simulink model "sldemo_fuelsys"  (R2024a)
settings: Solver=ode45  StartTime=0  StopTime=2000  FixedStep=0.001  RelTol=1e-5  AbsTol=1e-6
PostLoadFcn:
  | sldemo_fuelsys_data(bdroot,'initialize_data','orig','float');
model workspace (MAT data in the model file):
  PressEst = [0.806253176324 0.553142316929 0.37151500209 0.277667903103 0.220198954207 0.181288665766 0.153200000489 0.115431020872 0.0913067476324 0.0746519188607 0.0625231108324 0.0533383634277 ... (306 elements, 18x17)]
  PressVect = [0.05 0.1 0.15 0.2 0.25 0.3 0.35 0.4 0.45 0.5 0.55 0.6 ... (19 elements, 1x19)]
  PumpCon = [-0.0556348 -0.0022828 0.0256932 0.0435188 0.0562692 0.0661194857143 0.0741572 0.08697 0.0972452 0.106070342857 0.1139892 0.121303866667 ... (342 elements, 18x19)]
  RampRateKiX = [100 200 300 400 500 600]
  RampRateKiY = [0 0.2 0.4 0.6 0.8 1]
  RampRateKiZ = [0.012 0.024 0.036 0.048 0.06 0.072 0.024 0.048 0.072 0.096 0.12 0.144 ... (36 elements, 6x6)]
  SpeedEst = [471.837839721 550.80940091 777.559313277 1080.9243499 1418.36795322 1769.7468768 2125.37309264 2480.20345067 2831.37796793 3177.14006959 3516.32917143 4064.90417867 ... (323 elements, 17x19)]
  SpeedVect = [50 75 100 125 150 175 200 250 300 350 400 450 ... (18 elements, 1x18)]
  ThrotEst = [0 0 0 0 0 0 0 0 0 0 0 0 ... (342 elements, 18x19)]
  ThrotVect = [0 3 6 9 12 15 18 21 24 27 30 35 ... (17 elements, 1x17)]
  ego_sw = 1
  engine_speed = 300
  hys = 25
  map_sw = 1
  max_ego = 1.2
  max_press = 0.95
  max_speed = 628
  max_throt = 90
  min_press = 0.05
  min_speed = 50
  min_throt = 3
  speed_sw = 1
  st_range = 0.0001
  throttle_sw = 1
  zero_thresh = 250
undefined symbols (not defined in the file or in its folder): DiscIntNeverNeededParam, sld_FuelModes, sldvsubsys
libraries: simulink x4, simulink_extras x1
(part 2 of 2)

== system sldemo_fuelsys/fuel_rate_control/fuel_calc/switchable_compensation/disabled_mode ==
  note: Disabled Mode Fuel Mode
  Action Port : ActionPort  ActionPortLabel=default:
  shutoff : Constant  Value=0  OutDataTypeStr=Inherit: Inherit via back propagation
  fuel_rate : Outport  InitialOutput=0  VectorParamsAs1DForOutWhenUnconnected=off
  wires:
  shutoff/1 -> fuel_rate/1

== system sldemo_fuelsys/fuel_rate_control/fuel_calc/switchable_compensation/low_mode ==
  note: Low Mode Fuel Mode
  fb_correction : Inport
  ff_fuel_rate : Inport  Port=2
  Action Port : ActionPort  ActionPortLabel=case [ LOW ]:
  Discrete Filter : DiscreteFilter  Numerator=[8.7696 -8.5104]  Denominator=[1 -0.7408]  a0EqualsOne=on  RndMeth=Simplest  OutDataTypeStr=Inherit: Same as input
  Sum3 : Sum  OutDataTypeStr=s16En7  RndMeth=Simplest
  fuel_rate : Outport  InitialOutput=0  VectorParamsAs1DForOutWhenUnconnected=off
  wires:
  ff_fuel_rate/1 -> Sum3/2
  Discrete Filter/1 -> Sum3/1
  Sum3/1 -> fuel_rate/1
  fb_correction/1 -> Discrete Filter/1

== system sldemo_fuelsys/fuel_rate_control/fuel_calc/switchable_compensation/rich_mode ==
  note: Rich Mode Fuel Mode
  ff_fuel_rate : Inport
  fb_correction : Inport  Port=2
  Action Port : ActionPort  ActionPortLabel=case [ RICH ]:
  Discrete Filter : DiscreteFilter  Numerator=[0 0.2592]  Denominator=[1 -0.7408]  a0EqualsOne=on  RndMeth=Simplest  OutDataTypeStr=Inherit: Same as input
  Sum2 : Sum  OutDataTypeStr=s16En7  RndMeth=Simplest
  fuel_rate : Outport  InitialOutput=0  VectorParamsAs1DForOutWhenUnconnected=off
  wires:
  fb_correction/1 -> Sum2/2
  ff_fuel_rate/1 -> Sum2/1
  Sum2/1 -> Discrete Filter/1
  Discrete Filter/1 -> fuel_rate/1

== stateflow chart sldemo_fuelsys/fuel_rate_control/control_logic ==
  state O2 [parallel]
    settings: executionOrder=1  description=This state determines the validity of the exhaust gas oxygen sensor (EGO) data.
    state A
      du:
      es_o.ego = es_i.ego;
      state O2_warmup
        settings: description=The EGO sensor must come up to temperature before its data is reliable.
      state O2_normal
        settings: description=Normal EGO sensor operation gives a reliable indication of excess oxygen in the exhaust gas, from which air/fuel mixture can be inferred.
      state O2_failure
        settings: description=The EGO sensor has failed.
      (default) -> O2_warmup
      O2_warmup -> O2_normal : [after(480,tick)]
        settings: description=The value for sufficient warm up to operational temperature (nominally 4.8 seconds).
      O2_failure -> O2_normal : [es_i.ego < max_ego] / Fail.DEC;
      O2_normal -> O2_failure : [es_i.ego > max_ego] / Fail.INC;
        settings: description=The failure condition is indicated by excessive output voltage.
    (default) -> A
  state Pressure [parallel]
    settings: executionOrder=2  description=This state assesses the validity of the manifold absolute pressure (MAP) sensor.
    state normal
      du:
      es_o.map = es_i.map;
      settings: description=The manifold pressure sensor gives a reliable indication of absolute pressure (MAP).
    state fail
      du:
      es_o.map = map_estimate(es_i.speed, es_i.throttle);
      settings: description=The pressure sensor (manifold, or MAP) no longer produces reliable data.
    state map = map_estimate(speed, throttle) [function]
    (default) -> Pressure.normal
    Pressure.fail -> Pressure.normal : [es_i.map > min_press & ...
        | es_i.map < max_press] /
        | Fail.DEC;
    Pressure.normal -> Pressure.fail : [es_i.map > max_press | ...
        | es_i.map < min_press] /
        | Fail.INC;
  state Throttle [parallel]
    settings: executionOrder=3  description=This state determines the validity of the throttle sensor signal.
    state normal
      du:
      es_o.throttle = es_i.throttle;
      settings: description=The throttle sensor gives a reliable indication of the angle of the throttle plate.
    state fail
      du:
      es_o.throttle = throttle_estimate(es_i.speed,es_i.map);
      settings: description=Signal levels indicate that the throttle sensor data is no longer valid.
    state throttle = throttle_estimate(speed, map) [function]
    (default) -> Throttle.normal
    Throttle.fail -> Throttle.normal : [es_i.throttle >  min_throt & ...
        | es_i.throttle < max_throt] /
        | Fail.DEC;
    Throttle.normal -> Throttle.fail : [es_i.throttle> max_throt | ...
        | es_i.throttle < min_throt] /
        | Fail.INC;
      settings: description=A failure is indicated by data which is outside the expected range, typically due to an open or short circuit.
  state Speed [parallel]
    settings: executionOrder=4  description="This state infers the validity of the speed sensor data.  A failure is indicated by the presence of manifold vacuum at zero speed."
    state normal
      du:
      es_o.speed = es_i.speed;
      settings: description=The speed sensor data accurately represents the engine speed.
    state fail
      du:
      es_o.speed = speed_estimate(es_i.throttle, es_i.map);
      settings: description=The engine speed data is no longer available.
    state speed = speed_estimate(throttle, map) [function]
    (default) -> Speed.normal
    Speed.fail -> Speed.normal : [es_i.speed > 0C] /
        | Fail.DEC;
    Speed.normal -> Speed.fail : [es_i.speed == 0C & ...
        | es_i.map < zero_thresh] /
        | Fail.INC;
      settings: description="Loss of a reliable speed sensor signal will indicate zero speed.  This is deemed invalid when the manifold vacuum indicates otherwise."
  state Fail [parallel]
    settings: executionOrder=5  description=This state maintains a count of the number of sensors in failure mode.
    state Multi
      settings: description=This state represents any of the conditions in which more than one sensor is in failure mode.
      state Three
        settings: description=Three of the engine sensors have failed.
      state Four
        settings: description=All four of the engine sensors have failed.
      state Two
        settings: description=Two of the engine sensors have failed.
      Three -> Four [order 1] : INC
      Two -> Three [order 2] : INC
      Four -> Three : DEC
      Three -> Two [order 2] : DEC
    state One
      settings: description=One of the engine sensors has failed.
    state None
      settings: description=Zero failures; all sensors are operational.
    (default) -> None
    None -> One : INC
    One -> Two [order 1] : INC
    Two -> One [order 1] : DEC
    One -> None [order 2] : DEC
  state Fueling_Mode [parallel]
    settings: executionOrder=6  description=This state interprets the other states in the chart to directly control the fueling mode.
    state Fuel_Disabled
      en:
      fuel_mode = DISABLED;
      settings: description=The fuel is completely shut off while in this state.
      state Overspeed
        settings: description=The speed is dangerously high, so shut off the fuel.
      state Shutdown
        settings: description=Cut off system operation due to multiple sensor failures.
      Overspeed -> (junction 67) : [in(Speed.normal) & ...
          | es_i.speed < (max_speed - hys)]
      (junction 67) -> Shutdown [order 2] : [in(Fail.Multi)]
    state Running
      settings: description=The fuel is actively controlled while in this state.
      (history)
      state Low_Emissions
        en:
        fuel_mode = LOW;
        (history)
        state Warmup
          settings: description="The sensors are all operational, but the oxygen (EGO) sensor is warming up.  We'll target a stoichiometric ratio, nonetheless, but won't close the loop around exhaust gas oxygen."
        state Normal
          settings: description=All sensors are in correct operating modes, so effective closed-loop mixture control can be used.
        Warmup -> (junction 68) : [in(O2.A.O2_normal)]
        (junction 68) -> Normal [order 2]
      state Rich_Mixture
        en:
        fuel_mode = RICH;
        settings: description=This mode enriches the mixture, lowering the air/fuel ratio.
        state Single_Failure
          settings: description=Continue uninterrupted engine operation, but with a richer mixture.
      (junction 68) -> Single_Failure [order 1] : [in(Fail.One)]
      Normal -> Single_Failure : [in(Fail.One)]
      Single_Failure -> Normal : [in(Fail.None)]
    (default) -> Warmup : {es_o = es_i;}
      settings: description=Need to copy the sensors to the output on entry since the individual elements of the bus signal are only updated in the during function.
    Running -> Overspeed [order 2] : [es_i.speed > max_speed]
    (junction 67) -> Running [order 1] : [!in(Fail.Multi)]
    Running -> Shutdown [order 1] : enter(Fail.Multi)
    Shutdown -> Rich_Mixture : exit(Fail.Multi)
  data: speed function_input s16En3; throttle function_input s16En3; map function_output; speed function_input s16En3; map function_input u8En7; throttle function_output; throttle function_input s16En3; map function_input u8En7; speed function_output; es_o output EngSensors; O2_normal output boolean; max_ego parameter s16En7 [0..2]; max_press parameter u8En7 [0..2]; min_press parameter u8En7 [0..2]; min_throt parameter s16En3 [0..120]; max_throt parameter s16En3 [0..120]; zero_thresh parameter u8En7 [0..450]; max_speed parameter s16En3 [0..1000]; hys parameter s16En3 [0..1000]; es_i input EngSensors; fuel_mode output Enum: sld_FuelModes [1..3] =sld_FuelModes.LOW
  data es_o settings: description=Bus containing the sensor data.
  data max_ego settings: description=Parameter represents the upper end of the EGO sensor range.
  data max_press settings: description=Parameter represents the upper limt of valid pressure readings.
  data min_press settings: description=Parameter for the lower end of the valid pressure sensor range.
  data min_throt settings: description=Minimum valid throttle angle.
  data max_throt settings: description=Parameter to indicate the maximum valid throttle angle reading.
  data zero_thresh settings: description=Minimum manifold pressure expected at zero speed.
  data max_speed settings: description=Parameter for the upper end of the safe engine speed range.
  data hys settings: description=Hysteresis in the upper speed limit to avoid chatter at the threshold.
  data es_i settings: description=Bus containing the sensor data.
  data fuel_mode settings: description=Fuel control mode: LOW = stoichiometric mixture, RICH = rich mixture, DISABLED = shut down
  events: DEC local EITHER_EDGE_EVENT; INC local EITHER_EDGE_EVENT

== matlab function sldemo_fuelsys/Engine Gas Dynamics/Throttle & Manifold/Throttle/f(theta) ==
  data: u input; y output
function y = f(u)
%#codegen

y = 2.821 - 0.05231*u + 0.10299*u^2 - 0.00063*u^3;

== matlab function sldemo_fuelsys/Engine Gas Dynamics/Throttle & Manifold/Throttle/g(pratio) ==
  data: u input; y output
function y = g(u)
%#codegen

y = 2*sqrt(u - u^2);

== matlab function sldemo_fuelsys/Engine Gas Dynamics/Throttle & Manifold/Intake Manifold/MATLAB Function ==
  data: u1 input; y output; u2 input
function y = pumping(u1,u2)
%#codegen

y = -0.366 + 0.08979*u1*u2 - 0.0337*u2*u1^2 + 0.0001*u1*u2^2;

== matlab function sldemo_fuelsys/Engine Gas Dynamics/Mixing & Combustion/EGO Sensor ==
  data: u input; y output
function y = fcn(u)
%#codegen

y = (1-tanh(4*(u-14.6)))/2;
